simulink library "QuadRotor"  (R2018b)
settings: Solver=VariableStepAuto  StartTime=0.0  StopTime=10.0  RelTol=1e-3
undefined symbols (not defined in the file or in its folder): AERO, Clockwise, CONTROLLER, Counter, GEOMETRY, k_d_z, k_i_pitch, k_i_roll, k_i_yaw, k_i_z, k_p_pitch, k_p_roll, k_p_yaw, k_p_z, PROPULSION, SIMULATION, tFail, Ts
libraries: $bdroot x30, vrlib x5, aerolibutil x2, UWAerospaceBlockset_FlightParameters x2, UWAerospaceBlockset_Utilities x2, aerolibanimutils x1, aerolibobsolete x1, RCAM x1, aerolibadyn x1, UWAerospaceBlockset_EquationsOfMotion x1, UWAerospaceBlockset_Controllers x1, UWMiscBlockset x1
(part 1 of 2)
settings Model: Creator=Christopher  LastModifiedBy=admin

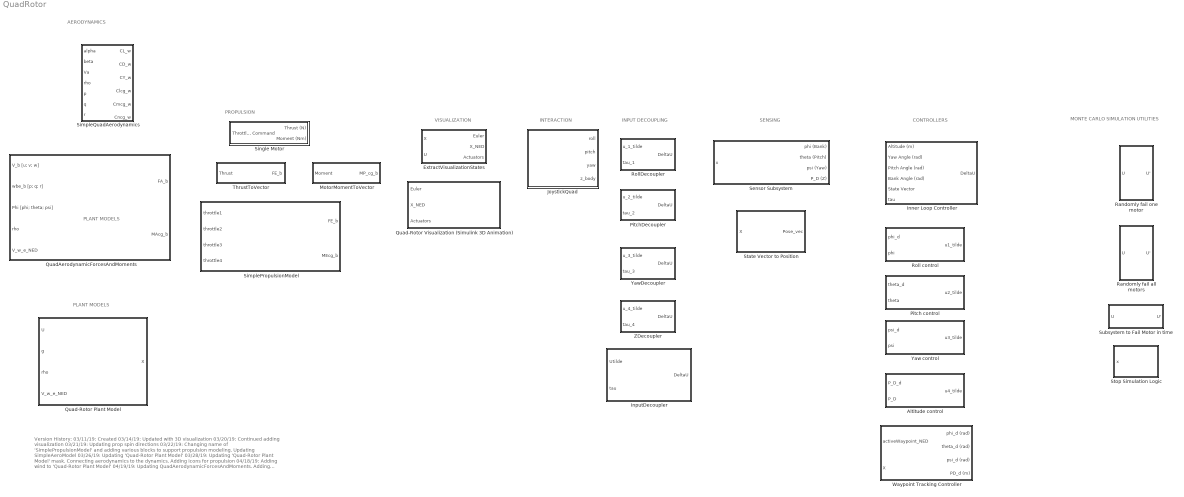
== system QuadRotor ==
  note: MONTE CARLO SIMULATION UTILITIES
  note: INTERACTION
  note: INPUT DECOUPLING
  note: PLANT MODELS
  note: Version History:
      | 03/11/19: Created
      | 03/14/19: Updated with 3D visualization
      | 03/20/19: Continued adding visualization
      | 03/21/19: Updating prop spin directions
      | 03/22/19: Changing name of 'SimplePropulsionModel' and adding various blocks to support propulsion modeling.  Updating SimpleAeroModel
      | 03/26/19: Updating 'Quad-Rotor Plant Model'
      | 03/28/19: Updating 'Quad-Rotor Plant Model' mask.  Connecting aerodynamics to the dynamics.  Adding icons for propulsion
      | 04/18/19: Adding wind to 'Quad-Rotor Plant Model'
      | 04/19/19: Updating QuadAerodynamicForcesAndMoments.  Adding decoupling input matrix
      | 04/27/19: Continued working InputDecoupler
      | 04/28/19: Changed order of InputDecoupler.  Added JoystickQuad
      | 04/29/19: Updating JoystickQuad
      | 05/07/19: Updated Inner Loop control units, added sensor subsystem
      | 05/14/19: Finalizing Inner Loop controllers
      | 05/21/19: Added Outer Loop Controller
      | 05/22/19: Renaming 'Outer Loop Controller' to 'Waypoint Tracking Controller'
      | 05/22/19: Edited Inner Loop control and Sensor Subsystem
      | 05/23/19: Added State Vector to Position
      | 06/03/19: Updating inner loop controllers to fix naive PID problems
      | 06/04/19: Updates to Inner Loop Controller interface
      | 06/09/19: Fixing various mistakes introduced by inexperienced developers.
      | 06/09/19: Added subsystem for randomly failing one motor with randomized time failure threshold
      | 06/12/19: Added subsystem for randomly failing all motors at a randomized time failure threshold
  note: VISUALIZATION
  note: CONTROLLERS
  note: PLANT MODELS
  note: PROPULSION
  note: AERODYNAMICS
  note: SENSING
  Altitude control : Subsystem  mask{k_p_z=k_p_z, k_i_z=k_i_z, k_d_z=k_d_z}
      mask prompts: k_p_z "Proportional gain for Z control"; k_i_z "Integral gain for Z control"; k_d_z "Derivative gain for Z control"
      mask help:
      | Control algorithm for Z control.
      |
      | INPUTS:
      |
      | - P_D_d: Desired height of COM in global frame
      | - P_D: Current height of COM in global frame
      |
      | OUTPUTS:
      |
      | - u2_tilde: Control input for Z control
  ExtractVisualizationStates : Subsystem
      mask help:
      | Extracts the relevant states and controls and repackages them so they can be used for visualization
      |
      |     X = [   u (m/s)
      |                v (m/s)
      |                w (m/s)
      |                p (rad/s)
      |                q (rad/s)
      |                r (rad/s)
      |                phi (bank angle: rad)
      |                theta (pitch angle: rad)
      |                psi (yaw angle: rad)
      |                P_N (position north (AKA X_e): m)
      |                P_E (position east (AKA Y_e): m)
      |                P_D (position down (AKA Z_e): m)
      |         ]
      |
      |     U = [	d_th1 (throttle 1 deflection: in range [0,1])
      |             	d_th2 (throttle 2 deflection: in range [0,1]
      | 	d_th3 (throttle 3 deflection: in range [0,1]
      | 	d_th4 (throttle 4 deflection: in range [0,1])
      |         ]
      |
      | INPUTS:
      | -X: 12x1 state vector as described above
      | -U: 4x1 control vector as described above
      |
      | OUTPUS
      | -Euler: 3x1 vector of [phi;theta;psi] (radians)
      | -X_NED: 3x1 vector of [P_N; P_E; P_D]  (m)
      | -Actuators: 4x1 vector in the range of [-1, 1] that denotes the relative speed of the 4 motors (see 'Quad-Rotor Visualization (Simulink 3D Animation) for more information)
      |
      | Created by Christopher Lum
      | lum@uw.edu
  Inner Loop Controller : Subsystem  mask{k_p_roll=k_p_roll, k_i_roll=k_i_roll, k_p_pitch=k_p_pitch, k_i_pitch=k_i_pitch, k_p_yaw=k_p_yaw, k_i_yaw=k_i_yaw, k_p_z=k_p_z, k_i_z=k_i_z, k_d_z=k_d_z}
      mask prompts: k_p_roll "Proportional Gain for Roll Control"; k_i_roll "Integral Gain for Roll Control"; k_p_pitch "Proportional Gain for Pitch Control"; k_i_pitch "Integral Gain for Pitch Control"; k_p_yaw "Proportional Gain for Yaw Control"; k_i_yaw "Integral Gain for Yaw Control"; k_p_z "Proportional Gain for Z control"; k_i_z "Integral Gain for Z control"; k_d_z "Derivative Gain for Z control"
      mask help:
      | Subsystem that compares current and reference values for altitude, yaw, pitch and roll values and converts it to control inputs to rotors.
      |
      | INPUTS:
      | -Altitude : scalar value transmitting desired altitude (m)
      | -Yaw Angle : scalar value transmitting desired yaw angle (radians)
      | -Pitch Angle : scalar value transmitting desired pitch angle (radians)
      | -Bank Angle : scalar value transmitting desired bank angle (radians)
      | -State Vector : 12x1 vector of current state [u ; v ; w ; p; q; r; phi ; theta ; psi ; P_N ; P_E ; P_D]
      | -tau: See 'InputDecoupler'
      |
      | OUTPUTS:
      | -DeltaU: 4X1 vector containing control signal pertubation to the four input signals
      |
      | Akshay Pai Raikar
      | apr244@uw.edu
      |
      | Updated by Christopher Lum
      | lum@uw.edu
  InputDecoupler : Subsystem
      mask help:
      | Decouples and remaps the inputs so attitude commands can be translated to motor commands.
      |
      | Utilde = [	roll command;
      | 	pitch command;
      | 	yaw command;
      | 	z command]
      |
      | tau = [	authority of roll command;
      | 	authority of pitch command;
      | 	authority of yaw command;
      | 	authority of z command]
      |
      | INPUTS:
      | Utilde: 4x1 vector in range [-1,1]
      | tau: 4x1 vector in range [0,1]
      |
      | OUTPUTS:
      | DeltaU: 4x1 vector in range [-1,1] that denotes how much to change each motor by
      |
      | Created by Christopher Lum
      | lum@uw.edu
  JoystickQuad : Subsystem  mask{joystickID=Joystick1, sample_time=SIMULATION.sample_time}
      mask prompts: joystickID "Joystick ID"; sample_time "Sample time (sec)"
      mask help:
      | Allows input from the joystick to be mapped to commands.
      |
      | INPUTS: -none
      |
      | OUTPUTS:
      | -roll:   command in the roll axis (in range [-1,1])
      | -pitch:  command in the pitch axis (in range [-1,1])
      | -yaw:    command in the yaw axis (in range [-1,1])
      | -z_body:  command in the z_body direction (in range [-1,1])
      mask TypeOptions joystickID: Joystick1 | Joystick2 | None
      mask Callback joystickID: animation_joystickID_CB(gcb)
      mask Display:
      | %Draw an icon
      | image('joystick.png')
  MotorMomentToVector : Subsystem  mask{direction=Clockwise}
      mask prompts: direction "Motor Spin Direction (when viewed from above)"
      mask help:
      | Converts the motor shaft toruqe/moment magnitude to a moment vector expressed in the body frame.  This assumes the motors are aligned perfectly with the z-axis and than the resulting moment due to the spinning prop is in the opposite direction of the propeller spin.
      |
      | INPUT:
      | Moment: The moment produced by the motor (Nm)
      |
      | OUTPUT:
      | M_P_cg_b: 3x1 moment vector aligned with body frame (Nm)
      mask TypeOptions direction: Clockwise | Counter-Clockwise
  Pitch control : Subsystem  mask{k_p_pitch=k_p_pitch, k_i_pitch=k_i_pitch}
      mask prompts: k_p_pitch "Proportional Gain for Pitch Control"; k_i_pitch "Integral Gain for Pitch Control"
      mask help:
      | Control algorithm for pitch control.
      |
      | INPUTS:
      |
      | - theta_d: Desired Theta angle value
      | - theta: Current theta angle value
      |
      | OUTPUTS:
      |
      | - u2_tilde: Control input for pitch control
  PitchDecoupler : Subsystem
      mask help:
      | Computes the changes in U that are can be used to create a pitch rate on the aircraft.
      |
      | INPUTS:
      | -u_2_tilde: pitch command in range [-1,1] (-1 = pitch down, +1 = pitch up)
      | -tau_2: control authority of pitch channel in range [0, 1]
      |
      | OUTPUTS:
      | -DeltaU: 4x1 vector denoting throttle commands in range [0,1] for the 4 motors
      |
      | Created by Christopher Lum
      | lum@uw.edu
  Quad-Rotor Plant Model : Subsystem  mask{CD=AERO.Static.CD, dMxbdp=AERO.Unsteady.dMxbdp, dMybdq=AERO.Unsteady.dMybdq, dMzbdr=AERO.Unsteady.dMzbdr, Tmax=PROPULSION.Tmax, Mmax=PROPULSION.Mmax, Xo=SIMULATION.X_0, m=GEOMETRY.mass, Ib=GEOMETRY.Ib, S=GEOMETRY.S, bref=GEOMETRY.bref, Xapt1=GEOMETRY.Xapt1, Yapt1=GEOMETRY.Yapt1, Zapt1=GEOMETRY.Zapt1, Xapt2=GEOMETRY.Xapt2, Yapt2=GEOMETRY.Yapt2, Zapt2=GEOMETRY.Zapt2, Xapt3=GEOMETRY.Xapt3, Yapt3=GEOMETRY.Yapt3, Zapt3=GEOMETRY.Zapt3, Xapt4=GEOMETRY.Xapt4, Yapt4=GEOMETRY.Yapt4, Zapt4=GEOMETRY.Zapt4}
      mask prompts: dMxbdp "dMx,b/dp"; dMybdq "dMy,b/dq"; dMzbdr "DMz,b/dr"; Tmax "Maximum thrust provided by one motor (N)"; Mmax "Maximum torque provided by one motor (Nm)"; Xo "Xo: initial condition"; m "Mass (kg)"; Ib "Inertia matrix (kg*m^2)"; S "Reference area (m^2)"; bref "Reference length (m)"; Xapt1 "x application point of thrust for motor 1 force in Fb (m)"; Yapt1 "y application point of thrust for motor 1 force in Fb (m)"; Zapt1 "z application point of thrust for motor 1 force in Fb (m)"; Xapt2 "x application point of thrust for motor 2 force in Fb (m)"; Yapt2 "y application point of thrust for motor 2 force in Fb (m)"; Zapt2 "z application point of thrust for motor 2 force in Fb (m)"; Xapt3 "x application point of thrust for motor 3 force in Fb (m)"; Yapt3 "y application point of thrust for motor 3 force in Fb (m)"; Zapt3 "z application point of thrust for motor 3 force in Fb (m)"; Xapt4 "x application point of thrust for motor 4 force in Fb (m)"; Yapt4 "y application point of thrust for motor 4 force in Fb (m)"; Zapt4 "z application point of thrust for motor 4 force in Fb (m)"
      mask help:
      | Implements a quad-rotor model using Simulink blocks.
      |
      | State vector X and input vector U is defined as
      |
      |     X = [   u (m/s)
      |                v (m/s)
      |                w (m/s)
      |                p (rad/s)
      |                q (rad/s)
      |                r (rad/s)
      |                phi (bank angle: rad)
      |                theta (pitch angle: rad)
      |                psi (yaw angle: rad)
      |                P_N (position north (AKA X_e): m)
      |                P_E (position east (AKA Y_e): m)
      |                P_D (position down (AKA Z_e): m)
      |         ]
      |
      |     U = [	d_th1 (throttle 1 deflection: in range [0,1])
      |             	d_th2 (throttle 2 deflection: in range [0,1]
      | 	d_th3 (throttle 3 deflection: in range [0,1]
      | 	d_th4 (throttle 4 deflection: in range [0,1])
      |         ]
      |
      | The constant wind field is defined as V_w_e_NED which is a 3x1 vector that denotes the wind w.r.t. to the fixed earth frame and expressed in the NED frame.  For example, if the wind is coming from the North (in other words it is blowing/moving to the South) at 10 m/s then
      |
      | 	V_w_e_NED = [-10;0;0]
      |
      | INPUT:  	U:      control vector
      |         	g:      gravity magnitude (typically 9.81)
      |         	rho:    density (kg/m^3)
      | 	V_w_e_NED:	3x1 vector denoting wind field
      |
      | OUTPUT: 	X:      state vector
      |
      | Created by Christopher Lum
      | lum@uw.edu
      mask DialogControl Container9 Prompt: Aero
      mask DialogControl Container22 Prompt: Static Aerodynamics
      mask DialogControl Container23 Prompt: Unsteady Aerodynamics
      mask DialogControl Container14 Prompt: Propulsion
      mask DialogControl Container16 Prompt: Simulation
      mask DialogControl Container18 Prompt: Environment
      mask DialogControl Container12 Prompt: Geometry
      mask DialogControl Container17 Prompt: Motor 1
      mask DialogControl Container19 Prompt: Motor 2
      mask DialogControl Container20 Prompt: Motor 3
      mask DialogControl Container21 Prompt: Motor 4
      mask Display:
      | %Use an image from the 'icons' folder
      | image('Inspire1.png')
  Quad-Rotor Visualization (Simulink 3D Animation) : Subsystem  mask{propAnimationScale=1, Ts=Ts}
      mask prompts: propAnimationScale "Prop animation scale factor"; Ts "Sample Time (sec)"
      mask help:
      | This is a visualization of a quad rotor rendered using the Simulink 3D environment.  This is based off the asbQuadCopter project (by MathWorks)
      |
      | Note: Simulink should open up the VRML sink and it should display the aircraft model in a separate window.  If this does not occur, you may need to look under the mask and through down through subsystems until you find the VR Sink block.  Double click on this block to open the aircraft animation window.
      |
      | Further note that Simulink may close the VRML sink the first time it is run (it may display a warning with verbiage about 'Virtual world has been closed from outside of Simulink.'.  If this occurs, simply repeat the procedure of looking under the mask and double clicking on the VR Sink.
      |
      | INPUTS:
      | -Euler: 3x1 vector of [phi;theta;psi] (radians)
      | -X_NED: 3x1 vector of [P_N; P_E; P_D]  (m)
      | -Actuators: 4x1 vector in the range of [-1, 1] that denotes the relative speed of the 4 motors.  The vector is in the order or [front right; front left; rear left; rear right].  The numbering and positive direction of each motor is defined in \\UWMatlab\UWMatlab\Simulink\UWAerospaceBlockset\AircraftModels\QuadRotor.nb.  Note that the propeller angular speed in the animation is not accurate, it is merely used to give a rough idea of the state of the motors.  As such, a value of +1 yields a rate that "looks good" in the animation.  A value of 0 corresponds to no spin.  You can  change the relative speed of the prop by changing the 'prop animation scale factor' (for example if you want the props to spin faster for a given actuator value, then increase the the scale factor to a value larger than 1).
      |
      | Christopher Lum
      | lum@uw.edu
      mask Display:
      | %Draw an icon
      | image('Parrot.png')
  QuadAerodynamicForcesAndMoments : Subsystem  mask{CD=AERO.Static.CD, dMxbdp=AERO.Unsteady.dMxbdp, dMybdq=AERO.Unsteady.dMybdq, dMzbdr=AERO.Unsteady.dMzbdr, S=GEOMETRY.S, bref=GEOMETRY.bref}
      mask prompts: dMxbdp "dMx,b/dp"; dMybdq "dMy,b/dq"; dMzbdr "DMz,b/dr"; S "Reference area (m^2)"; bref "Reference length (m)"
      mask help:
      | Aerodynamic forces and moments for a quad.
      |
      | INPUTS:
      | -V_b: 3x1 vector of [u;v;w] (m/s)
      | -wbe_b: 3x1 vector of [p;q;r] (rad/s)
      | -Phi: 3x1 vector of [phi;theta;psi] (rad)
      | -rho: scalar air density (kg/m^3)
      | -V_w_e_NED: 3x1 vector of wind velocity expressed in NED (m/s)
      |
      | OUTPUTS:
      | -FA_b: 3x1 vector of aerodynamic force in body axis (N)
      | -MAcg_b: 3x1 vector of aerodynamic moments in body axis about CG (Nm)
      |
      | Created by Christopher Lum
      | lum@uw.edu
      mask DialogControl Container2 Prompt: Static Aerodynamics
      mask DialogControl Container3 Prompt: Unsteady Aerodynamics
      mask DialogControl Container4 Prompt: Geometry
      mask Display:
      | %Draw an icon
      | image('QuadAeroCFD.png')
  Randomly fail all motors : Subsystem  mask{tFail=tFail}
      mask prompts: tFail "Randomized failure with respect to time lapsed in simulation"
      mask help: Subsystem which allows for failure of a one motor by setting a randomized failure time threshold.
  Randomly fail one motor : Subsystem  mask{tFail=tFail}
      mask prompts: tFail "Randomized failure with respect to time lapsed in simulation"
      mask help: Subsystem which allows for failure of a one motor by setting a randomized failure time threshold.
  Roll control : Subsystem  mask{k_p_roll=k_p_roll, k_i_roll=k_i_roll}
      mask prompts: k_p_roll "Proportional Gain for Roll Controller"; k_i_roll "Integrator Gain for Roll Control"
      mask help:
      | Control algorithm for roll control.
      |
      | INPUTS:
      |
      | - phi_d: Desired roll angle
      | - phi: Current roll angle
      |
      | OUTPUTS:
      |
      | - u1_tilde : Roll angle control input
      |
      | Akshay Pai Raikar
      | apr244@uw.edu
  RollDecoupler : Subsystem
      mask help:
      | Computes the changes in U that are can be used to create a roll rate on the aircraft.
      |
      | INPUTS:
      | -u_1_tilde: roll command in range [-1,1] (-1 = roll left, +1 = roll right)
      | -tau_1: control authority of roll channel in range [0, 1]
      |
      | OUTPUTS:
      | -DeltaU: 4x1 vector denoting throttle commands in range [0,1] for the 4 motors
      |
      | Created by Christopher Lum
      | lum@uw.edu
  Sensor Subsystem : Subsystem
  SimplePropulsionModel : Subsystem  mask{Tmax=0, Mmax=0, r1=0, r2=0, r3=0, r4=0}
      mask prompts: Tmax "Max thrust of single motor (N)"; Mmax "Max moment of single motor (Nm)"; r1 "Position vector of motor 1 (3x1) in Fb (m)"; r2 "Position vector of motor 2 (3x1) in Fb (m)"; r3 "Position vector of motor 3 (3x1) in Fb (m)"; r4 "Position vector of motor 4 (3x1) in Fb (m)"
      mask help:
      | This is a simple propulsion model for a quadrotor.
      |
      | See QuadRotor.nb for more information.
      mask Display: image('QuadPropulsion.png')
  SimpleQuadAerodynamics : Subsystem  mask{CD=AERO.Static.CD, dMxbdp=AERO.Unsteady.dMxbdp, dMybdq=AERO.Unsteady.dMybdq, dMzbdr=AERO.Unsteady.dMzbdr, S=GEOMETRY.S, bref=GEOMETRY.bref}
      mask prompts: dMxbdp "dMx,b/dp"; dMybdq "dMy,b/dq"; dMzbdr "DMz,b/dr"; S "Reference area (m^2)"; bref "Reference length (m)"
      mask help:
      | Simple aerodynamics for a quad.
      |
      | Note that this may have some discontinuities at zero airspeed.  This discontinuity is introduced to avoid NaN values in the output.
      |
      | INPUTS:
      | -alpha: angle of attack (rad)
      | -beta: angle of sideslip (rad)
      | -Va: airspeed (m/s)
      | -p: roll rate (rad/s)
      | -q: pitch rate (rad/s)
      | -r: yaw rate (rad/s)
      |
      | OUTPUTS:
      | -CL_w: coefficient of lift in wind axis
      | -CD_w: coefficient of drag in wind axis
      | -CY_w: coefficient of sideforce in wind axis
      | -Clac_w: coefficient of roll in wind axis
      | -Cmac_w: coefficient of pitch in wind axis
      | -Cnac_w: coefficient of yaw in wind axis
      mask DialogControl Container2 Prompt: Static Aerodynamics
      mask DialogControl Container3 Prompt: Unsteady Aerodynamics
      mask DialogControl Container4 Prompt: Geometry
  Single Motor : Subsystem  mask{Tmax=0, Mmax=0}
      mask prompts: Tmax "Maximum Thrust (N)"; Mmax "Maximum Moment (Nm)"
      mask help:
      | This block represents a simple model of a single engine.
      |
      | Note that this does not model the sign of the thrust and moment.  It merely calculates the magnitude.  Expressing these as vectors is done by other blocks (such as the 'SimplePropulsionModel' block.
      |
      | INPUT
      | -Throttle Command:  In range of [0,1]
      |
      | OUTPUT
      | -Thrust:  Resultant thrust generated by motor (N)
      | -Moment: Resultant moment generated by the motor (Nm)
  State Vector to Position : Subsystem
  Stop Simulation Logic : Subsystem
      mask help:
      | Stop the simulation when the aircraft hits the ground (altitude goes below 0).
      |
      | INPUT: X: state vector
      mask Display:
      | %Use icon from the 'icons' folder
      | image('Stop.png')
  "Subsystem to Fail Motor in time " : Subsystem  mask{tFail=0}
      mask prompts: tFail "Ramdomly initalized failure time"
  ThrustToVector : Subsystem
      mask help:
      | Converts the thrust magnitude to a force vector expressed in the body frame.  This assumes the motors are aligned perfectly with the z-axis and than a positive thust yields a force in the negative z-direction (this is the typical orientation of a quad rotor motor).
      |
      | INPUT:
      | Thrust: scalar magnitude of thrust (positive tends to lift up the vehicle) (N)
      |
      | OUTPUT:
      | FE_b: 3x1 force vector aligned with body frame (N)
  Waypoint Tracking Controller : Subsystem  mask{theta_forward=CONTROLLER.WaypointTrackingController.theta_forward}
      mask prompts: theta_forward "Pitch angle to induce Forward Motion"
      mask help:
      | Computes the required altitude, heading angle, pitch angle, and bank angle to track a specified waypoint.
      |
      | INPUTS:
      | -X_NED: 		3x1 vector of aircraft position expressed in NED frame (m)
      | -waypoint_NED: 	3x1 vector of waypoint location expressed in the NED frame (m)
      |
      | OUTPUTS:
      | phi_d:		desired bank angle to track waypoint (rad)
      | theta_d:		desired pitch angle to track waypoint (rad)
      | psi_d:		desired yaw angle to track waypoint (rad)
      | P_D_d:		desired altitude to track waypoint (m)
  Yaw control : Subsystem  mask{k_p_yaw=k_p_yaw, k_i_yaw=k_i_yaw}
      mask prompts: k_p_yaw "Proportional gain for Yaw Control"; k_i_yaw "Integral gain for Yaw Control"
      mask help:
      | Control algorithm for yaw control.
      |
      | INPUTS:
      |
      | - psi_d: Desired Theta angle value
      | - psi: Current theta angle value
      |
      | OUTPUTS:
      |
      | - u3_tilde: Control input for yaw control
  YawDecoupler : Subsystem
      mask help:
      | Computes the changes in U that are can be used to create a yaw rate on the aircraft.
      |
      | INPUTS:
      | -u_3_tilde: yaw command in range [-1,1] (-1 = yaw left, +1 = yaw right)
      | -tau_3: control authority of yaw channel in range [0, 1]
      |
      | OUTPUTS:
      | -DeltaU: 4x1 vector denoting throttle commands in range [0,1] for the 4 motors
      |
      | Created by Christopher Lum
      | lum@uw.edu
  ZDecoupler : Subsystem
      mask help:
      | Computes the changes in U that are can be used to create a change in z-position of the aircraft.
      |
      | Note that if the aircraft is level, this roughy translates into an altitude command (but -1 yields gaining altitude and +1 yields losing altitude).
      |
      | INPUTS:
      | -u_4_tilde: z command in range [-1,1] (-1 = negative z position (gain "altitude"), +1 = positive z position (lose "altitude")
      | -tau_4: control authority of z channel in range [0, 1]
      |
      | OUTPUTS:
      | -DeltaU: 4x1 vector denoting throttle commands in range [0,1] for the 4 motors
      |
      | Created by Christopher Lum
      | lum@uw.edu

== system QuadRotor/Altitude control ==
  note: Version History:
      | 05/07/19: Created
      | 05/14/19: Updated
      | 06/03/19: Switching to pseudo-derivative and adding integrator anti-windup
  P_D_d : Inport
  P_D : Inport  Port=2
  Sum : Sum  Inputs=|+-
  altitude to P_D : Gain  Gain=-1
  z controller : Subsystem
  u4_tilde : Outport
  wires:
  P_D/1 -> Sum/2
  z controller/1(u4_tilde) -> u4_tilde/1
  Sum/1 -> z controller/1(e)
  altitude to P_D/1 -> Sum/1
  P_D_d/1 -> altitude to P_D/1

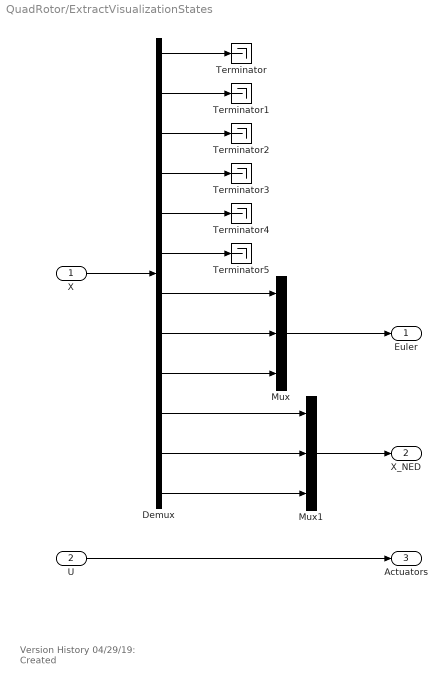
== system QuadRotor/ExtractVisualizationStates ==
  note: Version History
      | 04/29/19: Created
  X : Inport
  U : Inport  Port=2
  Demux : Demux  Outputs=12
  Mux : Mux  Inputs=3
  Mux1 : Mux  Inputs=3
  Terminator{,1..5} (6 alike) : Terminator
  Euler : Outport
  X_NED : Outport  Port=2
  Actuators : Outport  Port=3
  wires:
  X/1 -> Demux/1
  Demux/1 -> Terminator/1
  Demux/2 -> Terminator1/1
  Demux/3 -> Terminator2/1
  Demux/4 -> Terminator3/1
  Demux/5 -> Terminator4/1
  Demux/6 -> Terminator5/1
  Demux/7 -> Mux/1
  Demux/8 -> Mux/2
  Demux/9 -> Mux/3
  Demux/10 -> Mux1/1
  Demux/11 -> Mux1/2
  Demux/12 -> Mux1/3
  Mux/1 -> Euler/1
  Mux1/1 -> X_NED/1
  U/1 -> Actuators/1

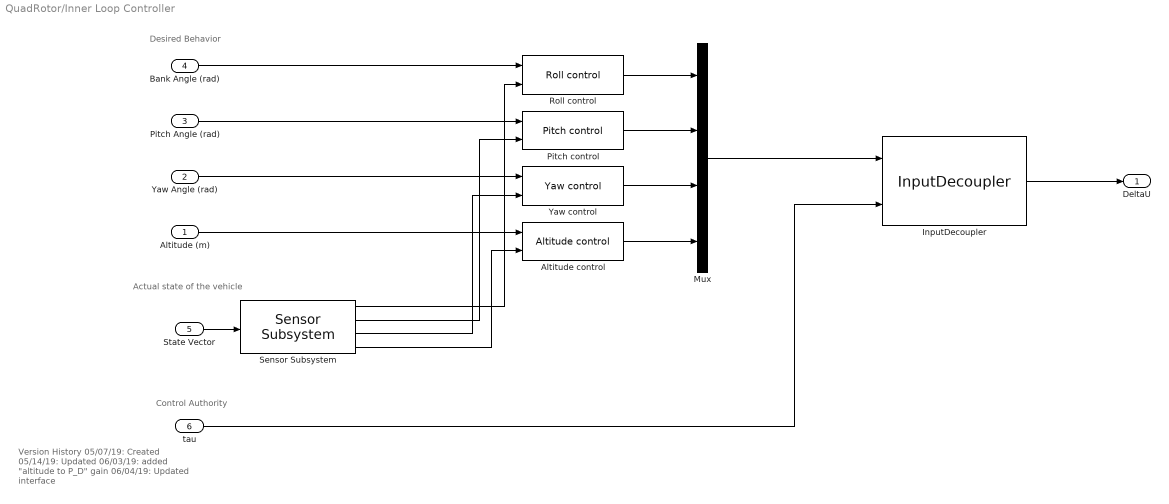
== system QuadRotor/Inner Loop Controller ==
  note: Control Authority
  note: Version History
      | 05/07/19: Created
      | 05/14/19: Updated
      | 06/03/19: added "altitude to P_D" gain
      | 06/04/19: Updated interface
  note: Actual state of the vehicle
  note: Desired Behavior
  Altitude (m) : Inport
  Yaw Angle (rad) : Inport  Port=2
  Pitch Angle (rad) : Inport  Port=3
  Bank Angle (rad) : Inport  Port=4
  " State Vector" : Inport  Port=5
  tau : Inport  Port=6
  Altitude control : $bdroot/Altitude control  k_p_z=k_p_z  k_i_z=k_i_z  k_d_z=k_d_z
  InputDecoupler : $bdroot/InputDecoupler
  Mux : Mux
  Pitch control : $bdroot/Pitch control  k_p_pitch=k_p_pitch  k_i_pitch=k_i_pitch
  Roll control : $bdroot/Roll control  k_p_roll=k_p_roll  k_i_roll=k_i_roll
  Sensor Subsystem : $bdroot/Sensor Subsystem  SystemSampleTime=-1
  Yaw control : $bdroot/Yaw control  k_p_yaw=k_p_yaw  k_i_yaw=k_i_yaw
  DeltaU : Outport
  wires:
  " State Vector"/1 -> Sensor Subsystem/1
  Bank Angle (rad)/1 -> Roll control/1
  Yaw Angle (rad)/1 -> Yaw control/1
  Roll control/1 -> Mux/1
  Pitch control/1 -> Mux/2
  Yaw control/1 -> Mux/3
  Mux/1 -> InputDecoupler/1
  tau/1 -> InputDecoupler/2
  Sensor Subsystem/1 -> Roll control/2
  Sensor Subsystem/2 -> Pitch control/2
  Sensor Subsystem/3 -> Yaw control/2
  InputDecoupler/1 -> DeltaU/1
  Altitude control/1 -> Mux/4
  Sensor Subsystem/4 -> Altitude control/2
  Pitch Angle (rad)/1 -> Pitch control/1
  Altitude (m)/1 -> Altitude control/1

== system QuadRotor/InputDecoupler ==
  note: Version History
      | 04/27/19: Created
      | 04/28/19: Changed order
  Utilde : Inport
  tau : Inport  Port=2
  Demux : Demux
  Demux1 : Demux
  PitchDecoupler : $bdroot/PitchDecoupler
  RollDecoupler : $bdroot/RollDecoupler
  Sum : Sum  Inputs=++++
  YawDecoupler : $bdroot/YawDecoupler
  ZDecoupler : $bdroot/ZDecoupler
  DeltaU : Outport
  wires:
  Utilde/1 -> Demux/1
  Demux/1 -> RollDecoupler/1
  Demux/2 -> PitchDecoupler/1
  Demux/3 -> YawDecoupler/1
  Demux/4 -> ZDecoupler/1
  tau/1 -> Demux1/1
  Demux1/1 -> RollDecoupler/2
  Demux1/2 -> PitchDecoupler/2
  Demux1/3 -> YawDecoupler/2
  Demux1/4 -> ZDecoupler/2
  YawDecoupler/1 -> Sum/3
  ZDecoupler/1 -> Sum/4
  Sum/1 -> DeltaU/1
  PitchDecoupler/1 -> Sum/2
  RollDecoupler/1 -> Sum/1

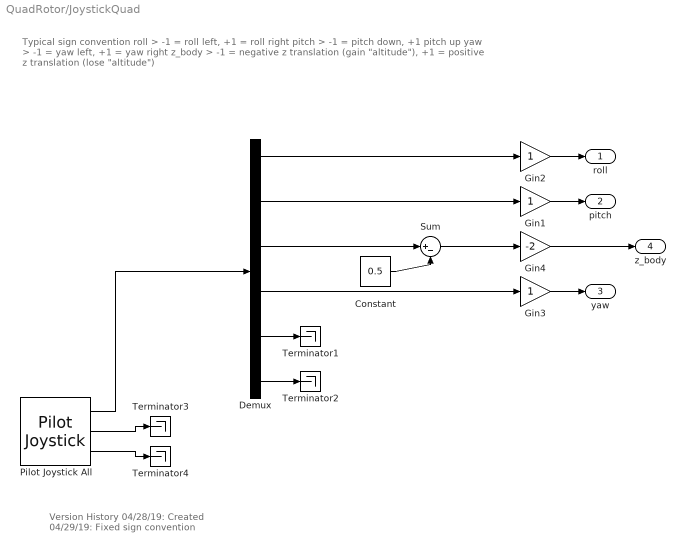
== system QuadRotor/JoystickQuad ==
  note: Version History
      | 04/28/19: Created
      | 04/29/19: Fixed sign convention
  note: Typical sign convention
      | roll        > -1 = roll left, +1 = roll right
      | pitch     > -1 = pitch down, +1 pitch up
      | yaw      > -1 = yaw left, +1 = yaw right
      | z_body > -1 = negative z translation (gain "altitude"), +1 = positive z translation (lose "altitude")
  Constant : Constant  Value=0.5
  Demux : Demux  Outputs=6
  Gin1 : Gain
  Gin2 : Gain
  Gin3 : Gain
  Gin4 : Gain  Gain=-2
  Pilot Joystick All : aerolibanimutils/Pilot Joystick  JoystickID=Joystick1  OutputConfiguration=AllOutputs  SampleTime=sample_time
  Sum : Sum  Inputs=|+-
  Terminator{1..4} (4 alike) : Terminator
  roll : Outport
  pitch : Outport  Port=2
  yaw : Outport  Port=3
  z_body : Outport  Port=4
  wires:
  Gin3/1 -> yaw/1
  Demux/4 -> Gin3/1
  Pilot Joystick All/3 -> Terminator4/1
  Pilot Joystick All/2 -> Terminator3/1
  Gin1/1 -> pitch/1
  Gin2/1 -> roll/1
  Demux/2 -> Gin1/1
  Demux/1 -> Gin2/1
  Demux/3 -> Sum/1
  Demux/6 -> Terminator2/1
  Demux/5 -> Terminator1/1
  Pilot Joystick All/1 -> Demux/1
  Constant/1 -> Sum/2
  Sum/1 -> Gin4/1
  Gin4/1 -> z_body/1

== system QuadRotor/MotorMomentToVector ==
  note: 1 = Clockwise
      | 2 = Counter-Clockwise
  note: Version History:
      | 03/22/19: Created
  Moment : Inport
  Constant : Constant  Value=0
  Constant1 : Constant  Value=direction
  Gain : Gain  Gain=-1
  Switch : Switch  Criteria=u2 > Threshold  Threshold=1
  Vector Concatenate : Concatenate  NumInputs=3
  MP_cg_b : Outport
  wires:
  Moment/1 -> Vector Concatenate/3
  Constant/1 -> Vector Concatenate/2, Vector Concatenate/1
  Constant1/1 -> Switch/2
  Vector Concatenate/1 -> Switch/1, Gain/1
  Gain/1 -> Switch/3
  Switch/1 -> MP_cg_b/1

== system QuadRotor/Pitch control ==
  note: Version History
      |
      | Created on :  05/07/19
      | Updated on : 05/14/19
  theta_d : Inport
  theta : Inport  Port=2
  Mux : Mux  Inputs=2
  Pitch Controller : Subsystem
  Pitch Signal Scope : Scope
  Sum : Sum  Inputs=|+-
  u2_tilde : Outport
  wires:
  theta/1 -> Mux/2, Sum/2
  theta_d/1 -> Mux/1, Sum/1
  Sum/1 -> Pitch Controller/1(e)
  Pitch Controller/1(u2_tilde) -> u2_tilde/1
  Mux/1 -> Pitch Signal Scope/1

== system QuadRotor/PitchDecoupler ==
  note: Version History
      | 04/27/19: Created
      | 04/28/19: Changed numbering
  u_2_tilde : Inport
  tau_2 : Inport  Port=2
  Gain : Gain  Gain=-1
  Mux : Mux
  Product : Product
  Product1 : Product
  Saturation : Saturate  UpperLimit=1  LowerLimit=0
  Saturation1 : Saturate  UpperLimit=1  LowerLimit=-1
  DeltaU : Outport
  wires:
  u_2_tilde/1 -> Saturation1/1
  tau_2/1 -> Saturation/1
  Product/1 -> Mux/2, Mux/1
  Gain/1 -> Product1/2
  Product1/1 -> Mux/4, Mux/3
  Saturation/1 -> Gain/1, Product/2
  Saturation1/1 -> Product/1, Product1/1
  Mux/1 -> DeltaU/1

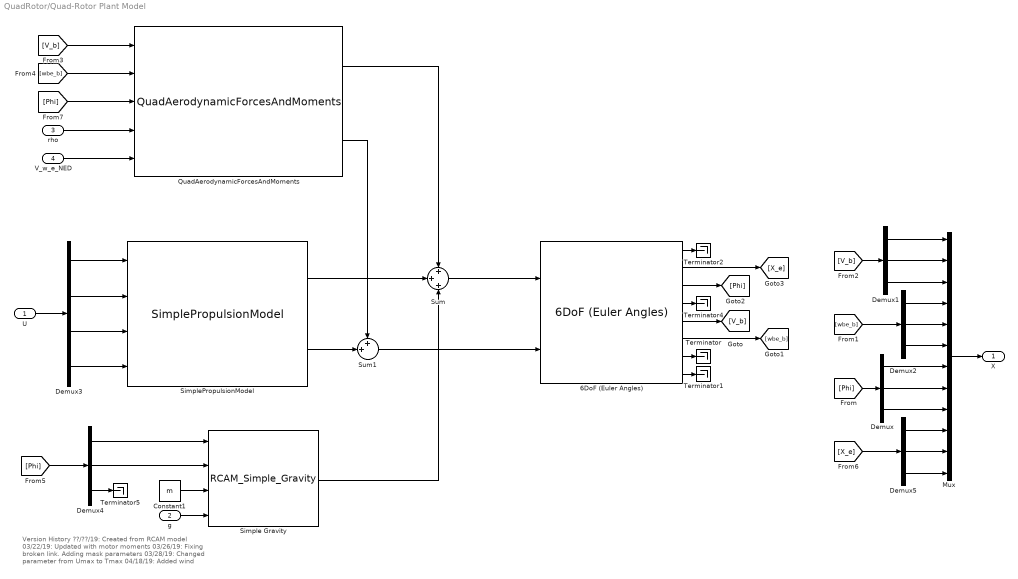
== system QuadRotor/Quad-Rotor Plant Model ==
  note: Version History
      | ??/??/19: Created from RCAM model
      | 03/22/19: Updated with motor moments
      | 03/26/19: Fixing broken link.  Adding mask parameters
      | 03/28/19: Changed parameter from Umax to Tmax
      | 04/18/19: Added wind
  U : Inport
  g : Inport  Port=2
  rho : Inport  Port=3
  V_w_e_NED : Inport  Port=4
  6DoF (Euler Angles) : aerolibobsolete/6DoF (Euler Angles)  units=Metric (MKS)  mtype=Fixed  rep=Euler Angles  xme_0=Xo(10:12)  Vm_0=Xo(1:3)  eul_0=Xo(7:9)  pm_0=Xo(4:6)  mass_0=m  mass_e=0.5  mass_f=2.0  inertia=Ib  inertia_e=eye(3)  inertia_f=2*eye(3)  k_quat=1.0
      settings: SourceProductName=Aerospace Blockset  SourceProductBaseCode=AE
  Constant1 : Constant  Value=m
  Demux{,1..2,4..5} (5 alike) : Demux  Outputs=3
  Demux3 : Demux
  Mux : Mux  Inputs=12
  QuadAerodynamicForcesAndMoments : $bdroot/QuadAerodynamicForcesAndMoments  CD=CD  dMxbdp=dMxbdp  dMybdq=dMybdq  dMzbdr=dMzbdr  S=S  bref=bref
  Simple Gravity : RCAM/RCAM_Simple_Gravity
  SimplePropulsionModel : $bdroot/SimplePropulsionModel  Tmax=Tmax  Mmax=Mmax  r1=[Xapt1; Yapt1; Zapt1]  r2=[Xapt2; Yapt2; Zapt2]  r3=[Xapt3; Yapt3; Zapt3]  r4=[Xapt4; Yapt4; Zapt4]
  Sum : Sum  Inputs=+|+|+
  Sum1 : Sum  Inputs=++|
  Terminator{,1..2,4..5} (5 alike) : Terminator
  X : Outport
  wires:
  Demux5/2 -> Mux/11
  Demux5/1 -> Mux/10
  Demux5/3 -> Mux/12
  [X_e] -> Demux5/1
  g/1 -> Simple Gravity/4
  Constant1/1 -> Simple Gravity/3
  Demux4/3 -> Terminator5/1
  Demux4/2 -> Simple Gravity/2
  Demux4/1 -> Simple Gravity/1
  [Phi] -> Demux4/1
  U/1 -> Demux3/1
  [V_b] -> Demux1/1
  [wbe_b] -> Demux2/1
  [Phi] -> Demux/1
  6DoF (Euler Angles)/3 -> [Phi]
  6DoF (Euler Angles)/6 -> [wbe_b]
  6DoF (Euler Angles)/5 -> [V_b]
  Mux/1 -> X/1
  6DoF (Euler Angles)/4 -> Terminator4/1
  6DoF (Euler Angles)/2 -> [X_e]
  6DoF (Euler Angles)/1 -> Terminator2/1
  6DoF (Euler Angles)/8 -> Terminator1/1
  6DoF (Euler Angles)/7 -> Terminator/1
  Demux2/3 -> Mux/6
  Demux2/2 -> Mux/5
  Demux2/1 -> Mux/4
  Demux1/3 -> Mux/3
  Demux1/2 -> Mux/2
  Demux1/1 -> Mux/1
  Demux/3 -> Mux/9
  Demux/2 -> Mux/8
  Demux/1 -> Mux/7
  Sum1/1 -> 6DoF (Euler Angles)/2
  Sum/1 -> 6DoF (Euler Angles)/1
  Simple Gravity/1 -> Sum/3
  Demux3/1 -> SimplePropulsionModel/1
  Demux3/2 -> SimplePropulsionModel/2
  Demux3/3 -> SimplePropulsionModel/3
  Demux3/4 -> SimplePropulsionModel/4
  SimplePropulsionModel/1 -> Sum/2
  SimplePropulsionModel/2 -> Sum1/2
  QuadAerodynamicForcesAndMoments/1 -> Sum/1
  QuadAerodynamicForcesAndMoments/2 -> Sum1/1
  [V_b] -> QuadAerodynamicForcesAndMoments/1
  [wbe_b] -> QuadAerodynamicForcesAndMoments/2
  rho/1 -> QuadAerodynamicForcesAndMoments/4
  [Phi] -> QuadAerodynamicForcesAndMoments/3
  V_w_e_NED/1 -> QuadAerodynamicForcesAndMoments/5

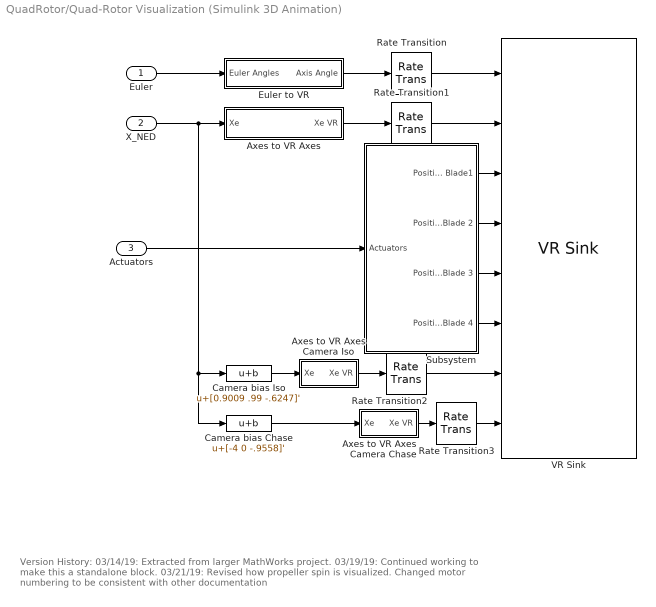
== system QuadRotor/Quad-Rotor Visualization (Simulink 3D Animation) ==
  note: Version History:
      | 03/14/19: Extracted from larger MathWorks project.
      | 03/19/19: Continued working to make this a standalone block.
      | 03/21/19: Revised how propeller spin is visualized.  Changed motor numbering to be consistent with other documentation
  Euler : Inport
  X_NED : Inport  Port=2
  Actuators : Inport  Port=3
  Axes to VR Axes : Subsystem
  Axes to VR Axes Camera Chase : Subsystem
  Axes to VR Axes Camera Iso : Subsystem
  Camera bias Chase : Bias  Bias=[-4 0 -.9558]'
  Camera bias Iso : Bias  Bias=[0.9009 .99 -.6247]'
  Euler to VR : Subsystem
  Rate Transition{,1..3} (4 alike) : RateTransition
  Subsystem : Subsystem
  VR Sink : vrlib/VR Sink  InstantiateOnLoad=on  SampleTime=12*Ts  ViewEnable=on  RemoteChange=off  RemoteView=off  FieldsWritten=QuadBody.rotation.4.1.1.double#QuadBody.translation.3.1.1.double#Blade1.rotation.4.1.1.double#Blade3.rotation.4.1.1.double#Blade2.rotation.4.1.1.double#Blade4.rotation.4.1.1.double#IsoNoRotation.position.3.1.1.double#OnQuadNoRotation.position.3.1.1.double  WorldFileName=asbQuadcopterWorld.wrl  AutoView=on  VideoDimensions=[]  AllowVariableSize=off  FigureProperties="{'Position', 'Name', 'Viewpoint', 'CameraBound', 'CameraDirection', 'CameraPosition', 'CameraUpVector', 'ZoomFactor', 'Antialiasing', 'Headlight', 'Lighting', 'NavPanel', 'Sound', 'StatusBar', 'Stereo3D', 'Stereo3DCameraOffset', 'Stereo3DHIT', 'ToolBar', 'Textures', 'Transparency', 'Triad', 'Wireframe', 'NavZones', 'NavMode', 'NavSpeed', 'CaptureFileFormat', 'CaptureFileName', 'Record2DCompressMethod', 'Record2DCompressQuality', 'Record2D', 'Record2DFileName', 'Record2DFPS'; [1.0000000000000000e+00   7.6000000000000000e+01   1.9200000000000000e+03   9.1300000000000000e+02], '', 'Isometric', 'on', [0.0000000000000000e+00   0.0000000000000000e+00  -1.0000000000000000e+00], [0.0000000000000000e+00   0.0000000000000000e+00   0.0000000000000000e+00], [0.0000000000000000e+00   1.0000000000000000e+00   0.0000000000000000e+00], [1.0000000000000000e+00], 'on', 'on', 'on', 'halfbar', 'on', 'on', 'off', [1.0000000149011612e-01], [0.0000000000000000e+00], 'on', 'on', 'on', 'none', 'off', 'off', 'fly', 'normal', 'tif', '%f_anim_%n.tif', 'auto', [7.5000000000000000e+01], 'off', '%f_anim_%n.avi', 'auto'}"
      settings: SourceProductBaseCode=VR
  wires:
  Camera bias Iso/1 -> Axes to VR Axes Camera Iso/1(Xe)
  Rate Transition1/1 -> VR Sink/2
  Axes to VR Axes/1(Xe VR) -> Rate Transition1/1
  Rate Transition/1 -> VR Sink/1
  Axes to VR Axes Camera Chase/1(Xe VR) -> Rate Transition3/1
  Rate Transition3/1 -> VR Sink/8
  X_NED/1 -> Camera bias Chase/1, Camera bias Iso/1, Axes to VR Axes/1(Xe)
  Camera bias Chase/1 -> Axes to VR Axes Camera Chase/1(Xe)
  Subsystem/3(Position Blade 3) -> VR Sink/5
  Subsystem/2(Position Blade 2) -> VR Sink/4
  Subsystem/1(Position Blade1) -> VR Sink/3
  Subsystem/4(Position Blade 4) -> VR Sink/6
  Euler to VR/1(Axis Angle) -> Rate Transition/1
  Axes to VR Axes Camera Iso/1(Xe VR) -> Rate Transition2/1
  Rate Transition2/1 -> VR Sink/7
  Actuators/1 -> Subsystem/1(Actuators)
  Euler/1 -> Euler to VR/1(Euler Angles)

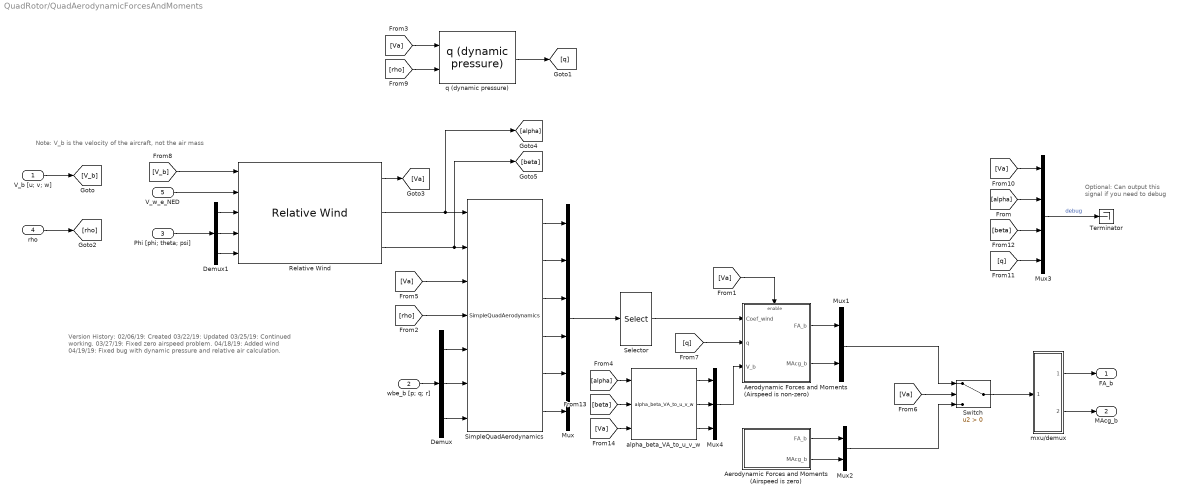
== system QuadRotor/QuadAerodynamicForcesAndMoments ==
  note: Optional: Can output this signal if you need to debug
  note: Note: V_b is the velocity of the aircraft, not the air mass
  note: Version History:
      | 02/06/19: Created
      | 03/22/19: Updated
      | 03/25/19: Continued working.
      | 03/27/19: Fixed zero airspeed problem.
      | 04/18/19: Added wind
      | 04/19/19: Fixed bug with dynamic pressure and relative air calculation.
  V_b [u; v; w] : Inport
  wbe_b [p; q; r] : Inport  Port=2
  Phi [phi; theta; psi] : Inport  Port=3
  rho : Inport  Port=4  Unit=kg/m^3
  V_w_e_NED : Inport  Port=5  Unit=kg/m^3
  Aerodynamic Forces and Moments (Airspeed is non-zero) : Subsystem
  Aerodynamic Forces and Moments (Airspeed is zero) : Subsystem
  Demux : Demux  Outputs=3
  Demux1 : Demux  Outputs=3
  Mux : Mux  Inputs=6
  Mux1 : Mux  Inputs=2
  Mux2 : Mux  Inputs=2
  Mux3 : Mux
  Mux4 : Mux  Inputs=3
  Relative Wind : UWAerospaceBlockset_EquationsOfMotion/Relative Wind
  Selector : Selector  InputPortWidth=6  IndexOptions=Index vector (dialog)  Indices=[2 3 1 4 5 6]  OutputSizes=1
  SimpleQuadAerodynamics : $bdroot/SimpleQuadAerodynamics  CD=CD  dMxbdp=dMxbdp  dMybdq=dMybdq  dMzbdr=dMzbdr  S=S  bref=bref
  Switch : Switch  Criteria=u2 > Threshold
  Terminator : Terminator
  alpha_beta_VA_to_u_v_w : UWAerospaceBlockset_FlightParameters/alpha_beta_VA_to_u_v_w
  mxu/demux : Subsystem
  q (dynamic pressure) : UWAerospaceBlockset_FlightParameters/q (dynamic pressure)
  FA_b : Outport
  MAcg_b : Outport  Port=2
  wires:
  V_b [u; v; w]/1 -> [V_b]
  Demux/1 -> SimpleQuadAerodynamics/5
  Demux/2 -> SimpleQuadAerodynamics/6
  Demux/3 -> SimpleQuadAerodynamics/7
  [rho] -> SimpleQuadAerodynamics/4
  rho/1 -> [rho]
  wbe_b [p; q; r]/1 -> Demux/1
  Relative Wind/2 -> [alpha], SimpleQuadAerodynamics/1
  Relative Wind/3 -> [beta], SimpleQuadAerodynamics/2
  SimpleQuadAerodynamics/1 -> Mux/1
  SimpleQuadAerodynamics/2 -> Mux/2
  SimpleQuadAerodynamics/3 -> Mux/3
  SimpleQuadAerodynamics/4 -> Mux/4
  SimpleQuadAerodynamics/5 -> Mux/5
  SimpleQuadAerodynamics/6 -> Mux/6
  Mux/1 -> Selector/1
  [Va] -> SimpleQuadAerodynamics/3
  [Va] -> Switch/2
  Selector/1 -> Aerodynamic Forces and Moments (Airspeed is non-zero)/1(Coef_wind)
  Aerodynamic Forces and Moments (Airspeed is non-zero)/1(FA_b) -> Mux1/1
  Aerodynamic Forces and Moments (Airspeed is non-zero)/2(MAcg_b) -> Mux1/2
  Aerodynamic Forces and Moments (Airspeed is zero)/1(FA_b) -> Mux2/1
  Aerodynamic Forces and Moments (Airspeed is zero)/2(MAcg_b) -> Mux2/2
  Mux2/1 -> Switch/3
  Mux1/1 -> Switch/1
  Switch/1 -> mxu/demux/1(" ")
  mxu/demux/1(FA_b) -> FA_b/1
  mxu/demux/2(MAcg_b) -> MAcg_b/1
  [Va] -> Aerodynamic Forces and Moments (Airspeed is non-zero)/Enable
  [q] -> Aerodynamic Forces and Moments (Airspeed is non-zero)/2(q)
  Mux4/1 -> Aerodynamic Forces and Moments (Airspeed is non-zero)/3(V_b)
  [V_b] -> Relative Wind/1
  V_w_e_NED/1 -> Relative Wind/2
  Demux1/1 -> Relative Wind/3
  Demux1/2 -> Relative Wind/4
  Demux1/3 -> Relative Wind/5
  Phi [phi; theta; psi]/1 -> Demux1/1
  Relative Wind/1 -> [Va]
  [rho] -> q (dynamic pressure)/2
  q (dynamic pressure)/1 -> [q]
  Mux3/1 -> Terminator/1  "debug"
  [Va] -> Mux3/1
  [Va] -> q (dynamic pressure)/1
  [alpha] -> alpha_beta_VA_to_u_v_w/1
  [beta] -> alpha_beta_VA_to_u_v_w/2
  [Va] -> alpha_beta_VA_to_u_v_w/3
  alpha_beta_VA_to_u_v_w/2 -> Mux4/2
  alpha_beta_VA_to_u_v_w/1 -> Mux4/1
  alpha_beta_VA_to_u_v_w/3 -> Mux4/3
  [alpha] -> Mux3/2
  [beta] -> Mux3/3
  [q] -> Mux3/4

== system QuadRotor/Randomly fail all motors ==
  U : Inport
  Demux : Demux
  Mux : Mux
  "Subsystem to Fail Motor 1 in time " : $bdroot/Subsystem to Fail Motor in time   tFail=0
  Subsystem to Fail Motor 2 in time 1 : $bdroot/Subsystem to Fail Motor in time   tFail=0
  Subsystem to Fail Motor 3 in time 2 : $bdroot/Subsystem to Fail Motor in time   tFail=0
  Subsystem to Fail Motor 4 in time 3 : $bdroot/Subsystem to Fail Motor in time   tFail=0
  U' : Outport
  wires:
  Mux/1 -> U'/1
  U/1 -> Demux/1
  "Subsystem to Fail Motor 1 in time "/1 -> Mux/1
  Demux/1 -> "Subsystem to Fail Motor 1 in time "/1
  Demux/2 -> Subsystem to Fail Motor 2 in time 1/1
  Subsystem to Fail Motor 2 in time 1/1 -> Mux/2
  Demux/3 -> Subsystem to Fail Motor 3 in time 2/1
  Subsystem to Fail Motor 3 in time 2/1 -> Mux/3
  Demux/4 -> Subsystem to Fail Motor 4 in time 3/1
  Subsystem to Fail Motor 4 in time 3/1 -> Mux/4

== system QuadRotor/Randomly fail one motor ==
  U : Inport
  Clock : Clock  Commented=on
  Constant : Constant  Commented=on  Value=0
  Demux : Demux
  Mux : Mux
  "Subsystem to Fail Motor in time " : $bdroot/Subsystem to Fail Motor in time   tFail=0
  Switch : Switch  Commented=on  Threshold=tFail
  U' : Outport
  wires:
  Mux/1 -> U'/1
  U/1 -> Demux/1
  Demux/2 -> Mux/2
  Demux/3 -> Mux/3
  Demux/4 -> Mux/4
  Clock/1 -> Switch/2
  Constant/1 -> Switch/1
  "Subsystem to Fail Motor in time "/1 -> Mux/1
  Demux/1 -> "Subsystem to Fail Motor in time "/1

== system QuadRotor/Roll control ==
  note: Version History:
      |
      | Created on: 05/07/19
      | Updated on: 05/14/19
  phi_d : Inport
  phi : Inport  Port=2
  Mux : Mux  Inputs=2
  Roll Controller : Subsystem
  Roll Signal Scope : Scope
  Sum : Sum  Inputs=|+-
  u1_tilde : Outport
  wires:
  Roll Controller/1(u1_tilde) -> u1_tilde/1
  Sum/1 -> Roll Controller/1(e)
  phi/1 -> Mux/2, Sum/2
  phi_d/1 -> Mux/1, Sum/1
  Mux/1 -> Roll Signal Scope/1

== system QuadRotor/RollDecoupler ==
  note: Version History
      | 04/27/19: Created
      | 04/28/19: Changed order
  u_1_tilde : Inport
  tau_1 : Inport  Port=2
  Gain : Gain  Gain=-1
  Mux : Mux
  Product : Product
  Product1 : Product
  Saturation : Saturate  UpperLimit=1  LowerLimit=0
  Saturation1 : Saturate  UpperLimit=1  LowerLimit=-1
  DeltaU : Outport
  wires:
  Mux/1 -> DeltaU/1
  Saturation1/1 -> Product1/1, Product/1
  Saturation/1 -> Product/2, Gain/1
  Gain/1 -> Product1/2
  tau_1/1 -> Saturation/1
  u_1_tilde/1 -> Saturation1/1
  Product/1 -> Mux/3, Mux/2
  Product1/1 -> Mux/4, Mux/1

== system QuadRotor/Sensor Subsystem ==
  x : Inport
  Demux : Demux  Outputs=12
  Terminator{,1..4,8..10} (8 alike) : Terminator
  phi (Bank) : Outport
  theta (Pitch) : Outport  Port=2
  psi (Yaw) : Outport  Port=3
  P_D (Z) : Outport  Port=4
  wires:
  Demux/1 -> Terminator/1
  Demux/5 -> Terminator4/1
  x/1 -> Demux/1
  Demux/2 -> Terminator1/1
  Demux/3 -> Terminator2/1
  Demux/4 -> Terminator3/1
  Demux/6 -> Terminator10/1
  Demux/7 -> phi (Bank)/1
  Demux/8 -> theta (Pitch)/1
  Demux/9 -> psi (Yaw)/1
  Demux/10 -> Terminator8/1
  Demux/11 -> Terminator9/1
  Demux/12 -> P_D (Z)/1

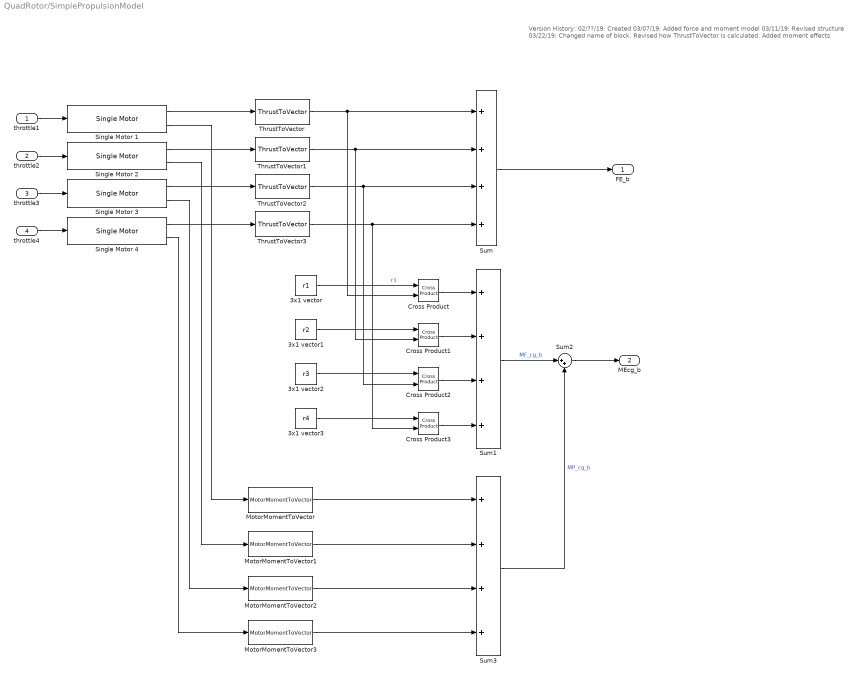
== system QuadRotor/SimplePropulsionModel ==
  note: Version History:
      | 02/??/19: Created
      | 03/07/19: Added force and moment model
      | 03/11/19: Revised structure
      | 03/22/19: Changed name of block.  Revised how ThrustToVector is calculated.  Added moment effects
  throttle1 : Inport
  throttle2 : Inport  Port=2
  throttle3 : Inport  Port=3
  throttle4 : Inport  Port=4
  3x1 vector : Constant  Value=r1
  3x1 vector1 : Constant  Value=r2
  3x1 vector2 : Constant  Value=r3
  3x1 vector3 : Constant  Value=r4
  Cross Product{,1..3} (4 alike) : vrlib/Utilities/Cross Product
      settings: SourceProductBaseCode=VR
  MotorMomentToVector : $bdroot/MotorMomentToVector  direction=Counter-Clockwise
  MotorMomentToVector1 : $bdroot/MotorMomentToVector  direction=Clockwise
  MotorMomentToVector2 : $bdroot/MotorMomentToVector  direction=Counter-Clockwise
  MotorMomentToVector3 : $bdroot/MotorMomentToVector  direction=Clockwise
  Single Motor {1..4} (4 alike) : $bdroot/Single Motor  Tmax=Tmax  Mmax=Mmax
  Sum : Sum  Inputs=++++
  Sum1 : Sum  Inputs=++++
  Sum2 : Sum  Inputs=|++
  Sum3 : Sum  Inputs=++++
  ThrustToVector{,1..3} (4 alike) : $bdroot/ThrustToVector
  FE_b : Outport
  MEcg_b : Outport  Port=2
  wires:
  3x1 vector3/1 -> Cross Product3/1
  3x1 vector2/1 -> Cross Product2/1
  3x1 vector1/1 -> Cross Product1/1
  Sum/1 -> FE_b/1
  ThrustToVector3/1 -> Sum/4, Cross Product3/2
  ThrustToVector2/1 -> Sum/3, Cross Product2/2
  ThrustToVector1/1 -> Sum/2, Cross Product1/2
  Single Motor 4/1 -> ThrustToVector3/1
  Single Motor 3/1 -> ThrustToVector2/1
  Single Motor 2/1 -> ThrustToVector1/1
  ThrustToVector/1 -> Sum/1, Cross Product/2
  Single Motor 1/1 -> ThrustToVector/1
  Cross Product3/1 -> Sum1/4
  Cross Product2/1 -> Sum1/3
  Cross Product1/1 -> Sum1/2
  Cross Product/1 -> Sum1/1
  3x1 vector/1 -> Cross Product/1  "r1"
  throttle4/1 -> Single Motor 4/1
  throttle3/1 -> Single Motor 3/1
  throttle2/1 -> Single Motor 2/1
  throttle1/1 -> Single Motor 1/1
  Sum1/1 -> Sum2/1  "MF_cg_b"
  Single Motor 1/2 -> MotorMomentToVector/1
  Single Motor 2/2 -> MotorMomentToVector1/1
  Single Motor 3/2 -> MotorMomentToVector2/1
  Single Motor 4/2 -> MotorMomentToVector3/1
  MotorMomentToVector2/1 -> Sum3/3
  MotorMomentToVector1/1 -> Sum3/2
  MotorMomentToVector3/1 -> Sum3/4
  MotorMomentToVector/1 -> Sum3/1
  Sum3/1 -> Sum2/2  "MP_cg_b"
  Sum2/1 -> MEcg_b/1

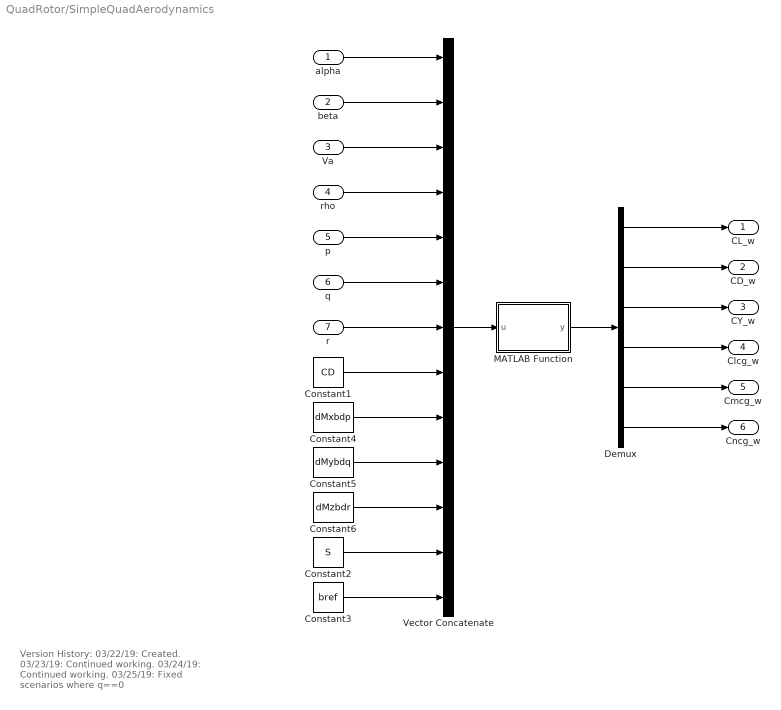
== system QuadRotor/SimpleQuadAerodynamics ==
  note: Version History:
      | 03/22/19: Created.
      | 03/23/19: Continued working.
      | 03/24/19: Continued working.
      | 03/25/19: Fixed scenarios where q==0
  alpha : Inport
  beta : Inport  Port=2
  Va : Inport  Port=3  Unit=kg/m^3
  rho : Inport  Port=4
  p : Inport  Port=5
  q : Inport  Port=6
  r : Inport  Port=7  Unit=kg/m^3
  Constant1 : Constant  Value=CD
  Constant2 : Constant  Value=S
  Constant3 : Constant  Value=bref
  Constant4 : Constant  Value=dMxbdp
  Constant5 : Constant  Value=dMybdq
  Constant6 : Constant  Value=dMzbdr
  Demux : Demux  Outputs=6
  MATLAB Function : MATLAB Function  TreatAsAtomicUnit=on
  Vector Concatenate : Concatenate  NumInputs=13
  CL_w : Outport
  CD_w : Outport  Port=2
  CY_w : Outport  Port=3
  Clcg_w : Outport  Port=4
  Cmcg_w : Outport  Port=5
  Cncg_w : Outport  Port=6
  wires:
  beta/1 -> Vector Concatenate/2
  Vector Concatenate/1 -> MATLAB Function/1(u)
  alpha/1 -> Vector Concatenate/1
  Va/1 -> Vector Concatenate/3
  MATLAB Function/1(y) -> Demux/1
  Demux/1 -> CL_w/1
  Demux/2 -> CD_w/1
  Demux/3 -> CY_w/1
  Demux/4 -> Clcg_w/1
  Demux/5 -> Cmcg_w/1
  Demux/6 -> Cncg_w/1
  rho/1 -> Vector Concatenate/4
  Constant4/1 -> Vector Concatenate/9
  Constant5/1 -> Vector Concatenate/10
  Constant6/1 -> Vector Concatenate/11
  p/1 -> Vector Concatenate/5
  q/1 -> Vector Concatenate/6
  r/1 -> Vector Concatenate/7
  Constant1/1 -> Vector Concatenate/8
  Constant2/1 -> Vector Concatenate/12
  Constant3/1 -> Vector Concatenate/13

== system QuadRotor/Single Motor ==
  note: Version History:
      | 03/07/19: Created
      | 03/22/19: Added moment
  Throttle Command : Inport
  Gain : Gain  Gain=Tmax
  Gain1 : Gain  Gain=Mmax
  Saturation : Saturate  UpperLimit=1  LowerLimit=0
  Thrust (N) : Outport
  Moment (Nm) : Outport  Port=2
  wires:
  Throttle Command/1 -> Saturation/1
  Saturation/1 -> Gain1/1, Gain/1
  Gain/1 -> Thrust (N)/1
  Gain1/1 -> Moment (Nm)/1

== system QuadRotor/State Vector to Position ==
  note: P_D
  note: P_E
  note: P_N
  note: Yaw
  note: Pitch
  note: Roll
  note: Version History:
      | 05/23/19: Created
      | 05/28/19: Modified to output Roll, Pitch, Yaw
      | 		  and P_N, P_E,P_D data
  note: Might need to replace with X_XYZ
  X : Inport
  Demux : Demux  Outputs=12
  Mux : Mux  Inputs=6
  Terminator{,1..4,10} (6 alike) : Terminator
  "Pose_vec " : Outport
  wires:
  X/1 -> Demux/1
  Demux/3 -> Terminator2/1
  Demux/4 -> Terminator3/1
  Demux/2 -> Terminator1/1
  Demux/1 -> Terminator/1
  Demux/5 -> Terminator4/1
  Demux/6 -> Terminator10/1
  Mux/1 -> "Pose_vec "/1
  Demux/7 -> Mux/1
  Demux/8 -> Mux/2
  Demux/9 -> Mux/3
  Demux/10 -> Mux/4
  Demux/11 -> Mux/5
  Demux/12 -> Mux/6

== system QuadRotor/Stop Simulation Logic ==
  x : Inport
  Constant : Constant
  Constant1 : Constant  Value=0
  Gain : Gain  Gain=-1
  Selector : Selector  InputPortWidth=12  IndexOptions=Index vector (dialog)  Indices=[12]  OutputSizes=1
  Stop Simulation : Stop
  Switch : Switch
  wires:
  x/1 -> Selector/1
  Selector/1 -> Gain/1  "PD"
  Gain/1 -> Switch/2  "h"
  Constant/1 -> Switch/3
  Constant1/1 -> Switch/1
  Switch/1 -> Stop Simulation/1

== system QuadRotor/Subsystem to Fail Motor in time  ==
  U : Inport
  Clock : Clock
  Constant : Constant  Value=0
  Switch : Switch  Threshold=tFail
  U' : Outport
  wires:
  Clock/1 -> Switch/2
  Constant/1 -> Switch/1
  U/1 -> Switch/3
  Switch/1 -> U'/1

== system QuadRotor/ThrustToVector ==
  note: Version History:
      | 03/11/19: Created
      | 03/22/19: Move to its own block.
  Thrust : Inport
  Constant : Constant  Value=0
  Gain1 : Gain  Gain=-1
  Vector Concatenate : Concatenate  NumInputs=3
  FE_b : Outport
  wires:
  Vector Concatenate/1 -> FE_b/1
  Constant/1 -> Vector Concatenate/1, Vector Concatenate/2
  Thrust/1 -> Gain1/1
  Gain1/1 -> Vector Concatenate/3

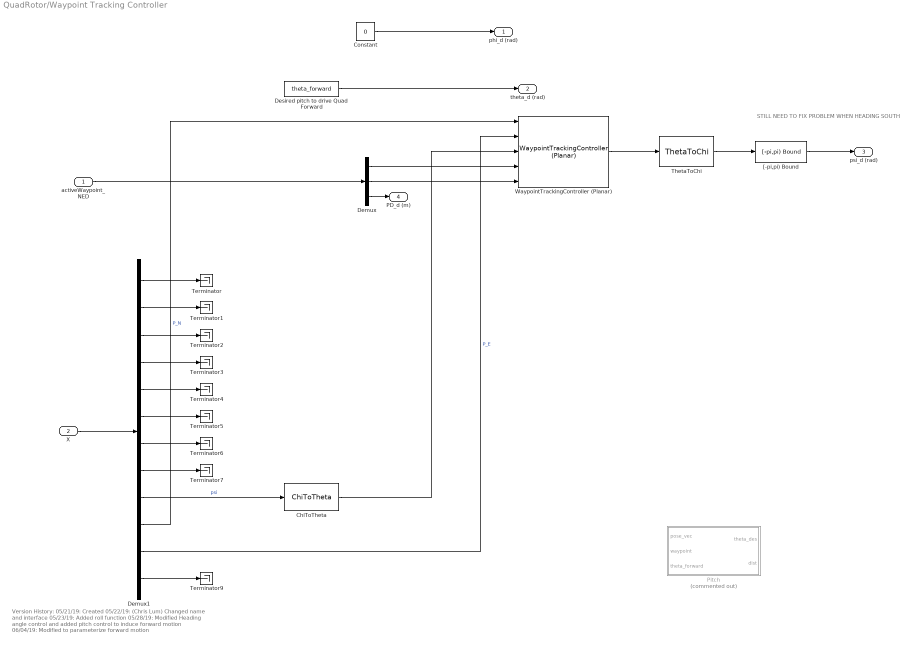
== system QuadRotor/Waypoint Tracking Controller ==
  note: STILL NEED TO FIX PROBLEM WHEN HEADING SOUTH
  note: Version History:
      |
      | 05/21/19: Created
      | 05/22/19: (Chris Lum) Changed name and interface
      | 05/23/19: Added roll function
      | 05/28/19: Modified Heading angle control and
      | 	         added pitch control to induce
      | 		  forward motion
      | 06/04/19: Modified to parameterize forward motion
  activeWaypoint_NED : Inport
  X : Inport  Port=2
  ChiToTheta : UWAerospaceBlockset_Utilities/ChiToTheta
  Constant : Constant  Value=0
  Demux : Demux  Outputs=3
  Demux1 : Demux  Outputs=12
  Desired pitch to drive Quad Forward : Constant  Value=theta_forward
  Pitch : MATLAB Function  Commented=on  TreatAsAtomicUnit=on
  Terminator{,1..7,9} (9 alike) : Terminator
  ThetaToChi : UWAerospaceBlockset_Utilities/ThetaToChi
  WaypointTrackingController (Planar) : UWAerospaceBlockset_Controllers/WaypointTrackingController (Planar)
  "[-pi,pi) Bound" : UWMiscBlockset/[-pi,pi) Bound  Description=|
      | Version History  
      |                  
      | 05/??/05: Created
  phi_d (rad) : Outport
  theta_d (rad) : Outport  Port=2
  psi_d (rad) : Outport  Port=3
  PD_d (m) : Outport  Port=4
  wires:
  activeWaypoint_NED/1 -> Demux/1
  Constant/1 -> phi_d (rad)/1
  X/1 -> Demux1/1
  Demux/1 -> WaypointTrackingController (Planar)/4
  Demux/2 -> WaypointTrackingController (Planar)/5
  WaypointTrackingController (Planar)/1 -> ThetaToChi/1
  Desired pitch to drive Quad Forward/1 -> theta_d (rad)/1
  Demux/3 -> PD_d (m)/1
  Demux1/1 -> Terminator/1
  Demux1/2 -> Terminator1/1
  Demux1/3 -> Terminator2/1
  Demux1/4 -> Terminator3/1
  Demux1/5 -> Terminator4/1
  Demux1/6 -> Terminator5/1
  Demux1/7 -> Terminator6/1
  Demux1/8 -> Terminator7/1
  Demux1/9 -> ChiToTheta/1  "psi"
  Demux1/12 -> Terminator9/1
  Demux1/10 -> WaypointTrackingController (Planar)/1  "P_N"
  Demux1/11 -> WaypointTrackingController (Planar)/2  "P_E"
  ChiToTheta/1 -> WaypointTrackingController (Planar)/3
  ThetaToChi/1 -> "[-pi,pi) Bound"/1
  "[-pi,pi) Bound"/1 -> psi_d (rad)/1

== system QuadRotor/Yaw control ==
  note: Version History
      |
      | Created on: 05/07/19
      | Updated on: 05/14/19
  psi_d : Inport
  psi : Inport  Port=2
  Mux : Mux  Inputs=2
  Sum : Sum  Inputs=|+-
  Yaw Controller : Subsystem
  Yaw Signal Scope : Scope
  u3_tilde : Outport
  wires:
  psi/1 -> Sum/2, Mux/2
  psi_d/1 -> Mux/1, Sum/1
  Yaw Controller/1(u3_tilde) -> u3_tilde/1
  Sum/1 -> Yaw Controller/1(e)
  Mux/1 -> Yaw Signal Scope/1

== system QuadRotor/YawDecoupler ==
  note: Version History
      | 04/27/19: Created
  u_3_tilde : Inport
  tau_3 : Inport  Port=2
  Gain : Gain  Gain=-1
  Mux : Mux
  Product : Product
  Product1 : Product
  Saturation : Saturate  UpperLimit=1  LowerLimit=0
  Saturation1 : Saturate  UpperLimit=1  LowerLimit=-1
  DeltaU : Outport
  wires:
  u_3_tilde/1 -> Saturation1/1
  tau_3/1 -> Saturation/1
  Gain/1 -> Product1/2
  Saturation/1 -> Gain/1, Product/2
  Saturation1/1 -> Product/1, Product1/1
  Mux/1 -> DeltaU/1
  Product/1 -> Mux/3, Mux/1
  Product1/1 -> Mux/4, Mux/2

== system QuadRotor/ZDecoupler ==
  note: Version History
      | 04/27/19: Created
  u_4_tilde : Inport
  tau_4 : Inport  Port=2
  Gain : Gain  Gain=-1
  Mux : Mux
  Product1 : Product
  Saturation : Saturate  UpperLimit=1  LowerLimit=0
  Saturation1 : Saturate  UpperLimit=1  LowerLimit=-1
  DeltaU : Outport
  wires:
  Mux/1 -> DeltaU/1
  Saturation1/1 -> Product1/1
  Saturation/1 -> Gain/1
  Gain/1 -> Product1/2
  tau_4/1 -> Saturation/1
  u_4_tilde/1 -> Saturation1/1
  Product1/1 -> Mux/1, Mux/2, Mux/4, Mux/3

== system QuadRotor/Altitude control/z controller ==
  note: Stable values:
      |
      | k_P --> 2
      | k_I --> 0.0034
      | k_D --> 1.22
  e : Inport
  Integrator : Integrator  LimitOutput=on  UpperSaturationLimit=30  LowerSaturationLimit=-30
  Pseudo-Derivative : TransferFcn  Numerator=[100 0]  Denominator=[1 100]
  Sum : Sum  Inputs=+++
  k_d_z : Gain  Gain=k_d_z
  k_i_z : Gain  Gain=k_i_z
  k_p_z : Gain  Gain=k_p_z
  u4_tilde : Outport
  wires:
  Sum/1 -> u4_tilde/1
  e/1 -> k_p_z/1, Pseudo-Derivative/1, Integrator/1
  k_p_z/1 -> Sum/2
  Integrator/1 -> k_i_z/1
  k_i_z/1 -> Sum/3
  k_d_z/1 -> Sum/1
  Pseudo-Derivative/1 -> k_d_z/1

== system QuadRotor/Pitch control/Pitch Controller ==
  note: Stable Values:
      |
      | k_P --> 0.86
      | k_I ---> 1.7
  e : Inport
  Gain : Gain  Gain=k_p_pitch
  Gain1 : Gain  Gain=k_i_pitch
  Integrator : Integrator
  Sum : Sum  Inputs=|++
  u2_tilde : Outport
  wires:
  e/1 -> Gain1/1, Gain/1
  Sum/1 -> u2_tilde/1
  Integrator/1 -> Sum/2
  Gain/1 -> Sum/1
  Gain1/1 -> Integrator/1
